simulink model "Assignment5Sim"  (R2020b)
settings: Solver=VariableStepAuto  StartTime=0.0  StopTime=3000  RelTol=1e-6
values from neighbouring files (symbols this model uses):
  E1 = 1    [Assignment5Mat.m]
  E2 = 1    [Assignment5Mat.m]
  freq1 = 5    [Assignment5Mat.m]
  freq2 = 1    [Assignment5Mat.m]
  gammaMat = [10 0 0 0 ... (first row only)    [Assignment5Mat.m]
  lambda = 2    [Assignment5Mat.m]
settings Model: Creator=Paolo  LastModifiedBy=Paolo

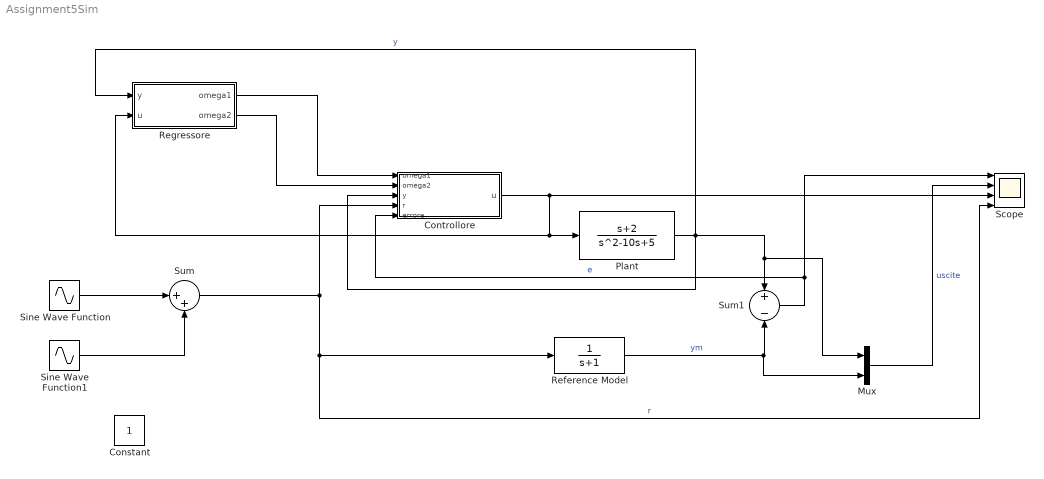
== system Assignment5Sim ==
  Constant : Constant
  Controllore : Subsystem
  Mux : Mux  Inputs=2
  Plant : TransferFcn  Numerator=[1 2]  Denominator=[1 -10 5]
  Reference Model : TransferFcn  Denominator=[1 1]
  Regressore : Subsystem
  Scope : Scope  NumInputPorts=4
  Sine Wave Function : Sin  Amplitude=E1  Frequency=freq1  SampleTime=0
  Sine Wave Function1 : Sin  Amplitude=E2  Frequency=freq2  SampleTime=0
  Sum : Sum  Inputs=|++
  Sum1 : Sum  Inputs=+|-
  wires:
  Plant/1 -> Controllore/3(y), Regressore/1(y), Mux/1, Sum1/1  "y"
  Sum/1 -> Scope/4, Reference Model/1, Controllore/4(r)  "r"
  Reference Model/1 -> Mux/2, Sum1/2  "ym"
  Sum1/1 -> Controllore/5(errore), Scope/1  "e"
  Mux/1 -> Scope/2  "uscite"
  Controllore/1(u) -> Plant/1, Regressore/2(u), Scope/3
  Regressore/1(omega1) -> Controllore/1(omega1)
  Regressore/2(omega2) -> Controllore/2(omega2)
  Sine Wave Function1/1 -> Sum/2
  Sine Wave Function/1 -> Sum/1

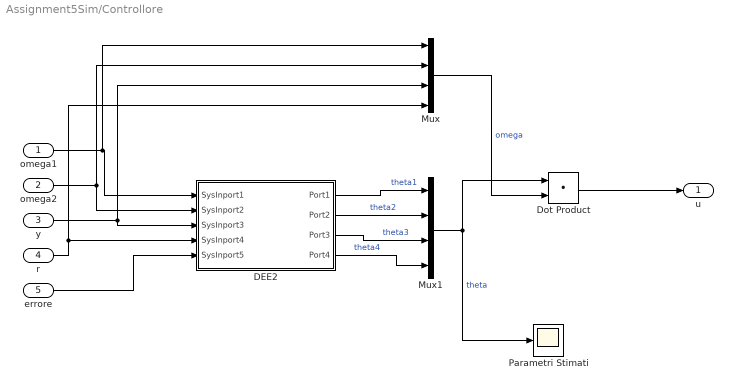
== system Assignment5Sim/Controllore ==
  omega1 : Inport
  omega2 : Inport  Port=2
  y : Inport  Port=3
  r : Inport  Port=4
  errore : Inport  Port=5
  DEE2 : Subsystem  mask(Differential Equation Editor (DEE)){}
      settings: OpenFcn=diffeqed
      mask Display: disp('Differential Equation\n Editor')
  Dot Product : DotProduct  InputSameDT=on  OutDataTypeStr=Inherit: Inherit via internal rule
  Mux : Mux
  Mux1 : Mux
  Parametri Stimati : Scope
  u : Outport
  wires:
  omega1/1 -> Mux/1, DEE2/1(SysInport1)
  omega2/1 -> Mux/2, DEE2/2(SysInport2)
  y/1 -> DEE2/3(SysInport3), Mux/3
  DEE2/1(Port1) -> Mux1/1  "theta1"
  DEE2/2(Port2) -> Mux1/2  "theta2"
  DEE2/3(Port3) -> Mux1/3  "theta3"
  r/1 -> DEE2/4(SysInport4), Mux/4
  errore/1 -> DEE2/5(SysInport5)
  DEE2/4(Port4) -> Mux1/4  "theta4"
  Dot Product/1 -> u/1
  Mux/1 -> Dot Product/2  "omega"
  Mux1/1 -> Parametri Stimati/1, Dot Product/1  "theta"

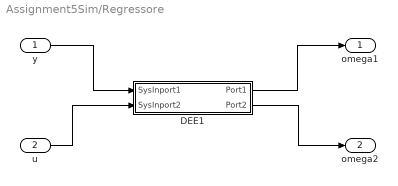
== system Assignment5Sim/Regressore ==
  y : Inport
  u : Inport  Port=2
  DEE1 : Subsystem  mask(Differential Equation Editor (DEE)){}
      settings: OpenFcn=diffeqed
      mask Display: disp('Differential Equation\n Editor')
  omega1 : Outport
  omega2 : Outport  Port=2
  wires:
  y/1 -> DEE1/1(SysInport1)
  u/1 -> DEE1/2(SysInport2)
  DEE1/1(Port1) -> omega1/1
  DEE1/2(Port2) -> omega2/1

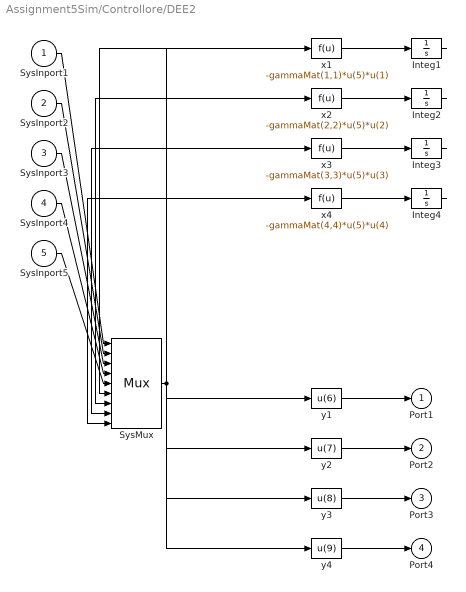
== system Assignment5Sim/Controllore/DEE2 ==
  SysInport1 : Inport
  SysInport2 : Inport  Port=2
  SysInport3 : Inport  Port=3
  SysInport4 : Inport  Port=4
  SysInport5 : Inport  Port=5
  Integ{1..4} (4 alike) : Integrator
  SysMux : Mux  Inputs=9
  x1 : Fcn  Expr=-gammaMat(1,1)*u(5)*u(1)
  x2 : Fcn  Expr=-gammaMat(2,2)*u(5)*u(2)
  x3 : Fcn  Expr=-gammaMat(3,3)*u(5)*u(3)
  x4 : Fcn  Expr=-gammaMat(4,4)*u(5)*u(4)
  y1 : Fcn  Expr=u(6)
  y2 : Fcn  Expr=u(7)
  y3 : Fcn  Expr=u(8)
  y4 : Fcn  Expr=u(9)
  Port1 : Outport
  Port2 : Outport  Port=2
  Port3 : Outport  Port=3
  Port4 : Outport  Port=4
  wires:
  SysInport1/1 -> SysMux/1
  SysInport2/1 -> SysMux/2
  SysInport3/1 -> SysMux/3
  SysInport4/1 -> SysMux/4
  SysInport5/1 -> SysMux/5
  SysMux/1 -> x1/1, x2/1, x3/1, x4/1, y1/1, y2/1, y3/1, y4/1
  x1/1 -> Integ1/1
  Integ1/1 -> SysMux/6
  x2/1 -> Integ2/1
  Integ2/1 -> SysMux/7
  x3/1 -> Integ3/1
  Integ3/1 -> SysMux/8
  x4/1 -> Integ4/1
  Integ4/1 -> SysMux/9
  y1/1 -> Port1/1
  y2/1 -> Port2/1
  y3/1 -> Port3/1
  y4/1 -> Port4/1

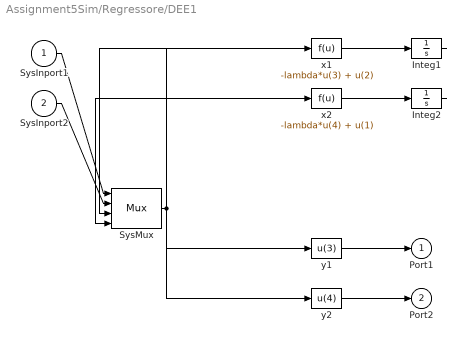
== system Assignment5Sim/Regressore/DEE1 ==
  SysInport1 : Inport
  SysInport2 : Inport  Port=2
  Integ1 : Integrator
  Integ2 : Integrator
  SysMux : Mux
  x1 : Fcn  Expr=-lambda*u(3) + u(2)
  x2 : Fcn  Expr=-lambda*u(4) + u(1)
  y1 : Fcn  Expr=u(3)
  y2 : Fcn  Expr=u(4)
  Port1 : Outport
  Port2 : Outport  Port=2
  wires:
  SysInport1/1 -> SysMux/1
  SysInport2/1 -> SysMux/2
  SysMux/1 -> x1/1, x2/1, y1/1, y2/1
  x1/1 -> Integ1/1
  Integ1/1 -> SysMux/3
  x2/1 -> Integ2/1
  Integ2/1 -> SysMux/4
  y1/1 -> Port1/1
  y2/1 -> Port2/1
